simulink model "den1"  (R2018a)
settings: Solver=VariableStepAuto  StartTime=0.0  StopTime=100  RelTol=1e-3
settings Model: Creator=Halil Temurtaş  LastModifiedBy=Halil Temurtaş
settings SolverCC: AlgebraicLoopSolver=LineSearch

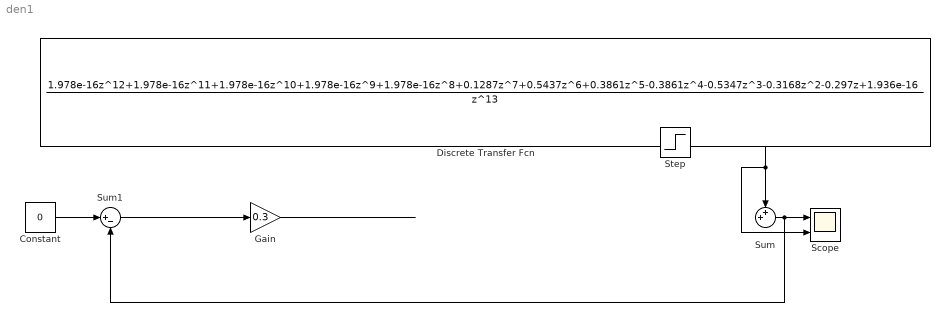
== system den1 ==
  Constant : Constant  Value=0
  Discrete Transfer Fcn : DiscreteTransferFcn  Numerator=[1.978e-16 1.978e-16 1.978e-16 1.978e-16 1.978e-16 0.1287 0.5437 0.3861 -0.3861 -0.5347 -0.3168 -0.297 1.936e-16]  Denominator=[1 0 0 0 0 0 0 0 0 0 0 0 0 0 ]
  Gain : Gain  Gain=0.3
  Scope : Scope  NumInputPorts=2
  Step : Step  SampleTime=0
  Sum : Sum  Inputs=++|
  Sum1 : Sum  Inputs=|+-
  wires:
  Gain/1 -> ?
  ? -> Sum/2
  Step/1 -> Scope/2, Sum/1
  Sum1/1 -> Gain/1
  Constant/1 -> Sum1/1
  Sum/1 -> Sum1/2, Scope/1
